simulink model "magball"  (R2018a)
settings: Solver=VariableStepAuto  StartTime=0.0  StopTime=10.0  RelTol=1e-3
settings Model: Creator=rosanal2  LastModifiedBy=rosanal2

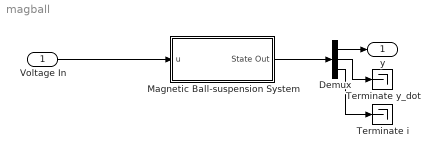
== system magball ==
  Voltage In : Inport
  Demux : Demux  Outputs=3
  Magnetic Ball-suspension System : Subsystem
  Terminate i : Terminator
  Terminate y_dot : Terminator
  y : Outport
  wires:
  Voltage In/1 -> Magnetic Ball-suspension System/1(u)
  Demux/1 -> y/1
  Demux/2 -> Terminate y_dot/1
  Demux/3 -> Terminate i/1
  Magnetic Ball-suspension System/1(State Out) -> Demux/1

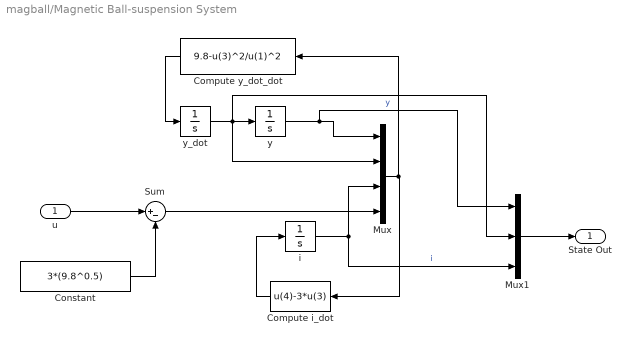
== system magball/Magnetic Ball-suspension System ==
  u : Inport
  Compute i_dot : Fcn  Expr=u(4)-3*u(3)
  Compute y_dot_dot : Fcn  Expr=9.8-u(3)^2/u(1)^2
  Constant : Constant  Value=3*(9.8^0.5)
  Mux : Mux
  Mux1 : Mux  Inputs=3
  Sum : Sum  Inputs=|+-
  i : Integrator  InitialCondition=sqrt(9.8)
  y : Integrator  InitialCondition=1
  y_dot : Integrator
  State Out : Outport
  wires:
  Mux1/1 -> State Out/1
  u/1 -> Sum/1
  Mux/1 -> Compute y_dot_dot/1, Compute i_dot/1
  Compute i_dot/1 -> i/1
  i/1 -> Mux1/3, Mux/3  "i"
  y_dot/1 -> Mux1/2, Mux/2, y/1
  Compute y_dot_dot/1 -> y_dot/1
  y/1 -> Mux1/1, Mux/1  "y"
  Sum/1 -> Mux/4
  Constant/1 -> Sum/2
